simulink model "mDriverSimpleTest"  (R2019b)
settings: Solver=ode4  StartTime=0  StopTime=2474  FixedStep=0.01  MaxStep=.01  RelTol=1e-3
libraries: VsrLibDriver x1, VsrLibDriveCycleSrc x1, autolibshared x1
settings Model: DataDictionary=DdDriverLongTest.sldd  SimulationMode=accelerator  PauseTimes=70  Creator=9bt  LastModifiedBy=4qz

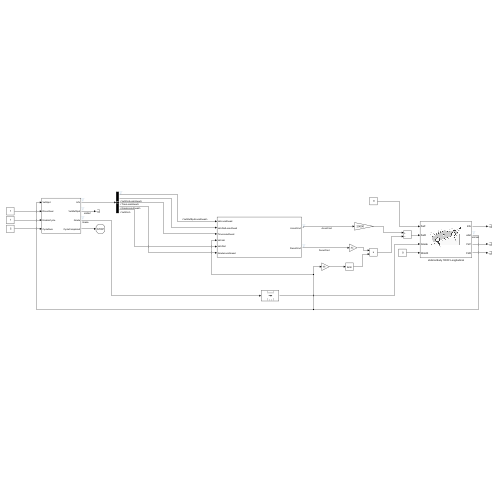
[thumbnail: Simulink's stored preview of the top-level diagram]
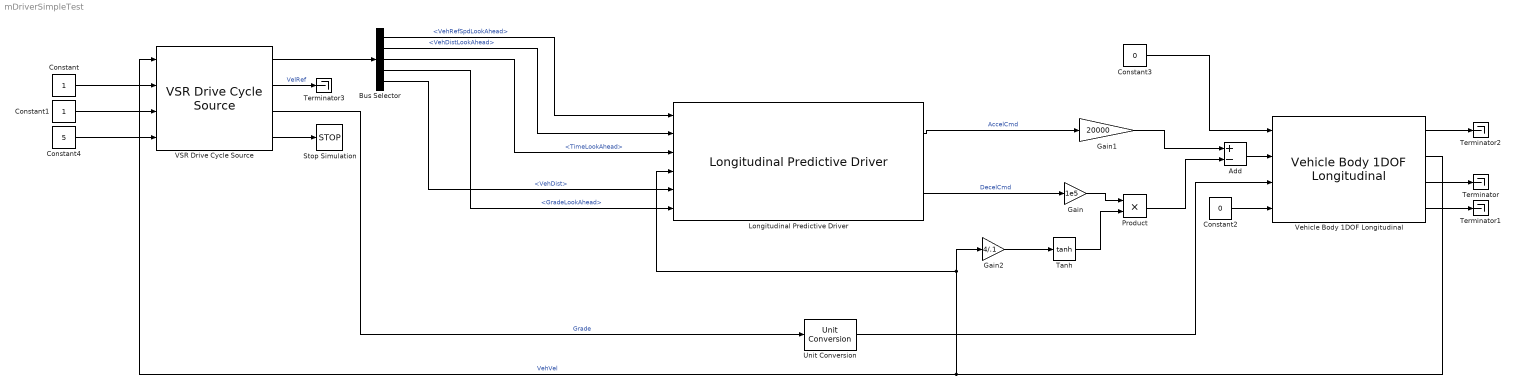
== system mDriverSimpleTest ==
  Add : Sum  Inputs=+-
  Bus Selector : BusSelector  OutputSignals=VehRefSpdLookAhead,VehDistLookAhead,TimeLookAhead,GradeLookAhead,VehDist
  Constant : Constant
  Constant1 : Constant
  Constant2 : Constant  Value=0
  Constant3 : Constant  Value=0
  Constant4 : Constant  Value=5
  Gain : Gain  Gain=1e5
  Gain1 : Gain  Gain=20000
  Gain2 : Gain  Gain=4/.1
  Longitudinal Predictive Driver : VsrLibDriver/Longitudinal Predictive Driver  VehMass=1500  aR=200  bR=2.5  cR=0.5  MaxAccelFrcSpdBpts=[ 10, 100 ]  MaxAccelFrcTbl=[ 10000, 10000 ]  AccelPdlBpts=[ 0, 1 ]  AccelPdlTbl=[ 0, 1 ]  BrakePdlBpts=[ 0, 1 ]  BrakeFrcTbl=[ 0, 1e5 ]  SmoothTimeAvg=.5  VelThresh=.1  PdlRateLimitWeight=.1  DistOptWeight=100  NumOptimIters=20  g=9.81
  Product : Product
  Stop Simulation : Stop
  Tanh : Trigonometry  Operator=tanh
  Terminator{,1..3} (4 alike) : Terminator
  Unit Conversion : UnitConversion
  VSR Drive Cycle Source : VsrLibDriveCycleSrc/VSR Drive Cycle Source  DistCompensationCheckbox=off  DriveCycleStructArray=VsrDriveCycleStructArray  TimeLookAhead=LookAheadTime
  Vehicle Body 1DOF Longitudinal : autolibshared/Vehicle Body 1DOF Longitudinal  VariantControl=SL  extFMode=off  extMMode=off  extTamb=off  wind3D=off  aMode=1  NF=2  NR=2  m=1500  a=1.4  b=1.8  h=.35  Cd=.3  Cl=0  Cpm=0  Af=4  x_o=0  xdot_o=0  Pabs=101325  T=273  g=9.81
  wires:
  Bus Selector/1 -> Longitudinal Predictive Driver/1  "<VehRefSpdLookAhead>"
  Constant2/1 -> Vehicle Body 1DOF Longitudinal/4
  Vehicle Body 1DOF Longitudinal/2 -> VSR Drive Cycle Source/1, Longitudinal Predictive Driver/4, Gain2/1  "VehVel"
  Vehicle Body 1DOF Longitudinal/3 -> Terminator/1
  Vehicle Body 1DOF Longitudinal/4 -> Terminator1/1
  Unit Conversion/1 -> Vehicle Body 1DOF Longitudinal/3
  VSR Drive Cycle Source/3 -> Unit Conversion/1  "Grade"
  Vehicle Body 1DOF Longitudinal/1 -> Terminator2/1
  Constant3/1 -> Vehicle Body 1DOF Longitudinal/1
  Add/1 -> Vehicle Body 1DOF Longitudinal/2
  Product/1 -> Add/2
  Gain1/1 -> Add/1
  Gain/1 -> Product/1
  Tanh/1 -> Product/2
  Gain2/1 -> Tanh/1
  Longitudinal Predictive Driver/1 -> Gain1/1  "AccelCmd"
  Longitudinal Predictive Driver/2 -> Gain/1  "DecelCmd"
  VSR Drive Cycle Source/2 -> Terminator3/1  "VelRef"
  VSR Drive Cycle Source/4 -> Stop Simulation/1
  VSR Drive Cycle Source/1 -> Bus Selector/1
  Constant1/1 -> VSR Drive Cycle Source/3
  Constant/1 -> VSR Drive Cycle Source/2
  Constant4/1 -> VSR Drive Cycle Source/4
  Bus Selector/2 -> Longitudinal Predictive Driver/2  "<VehDistLookAhead>"
  Bus Selector/3 -> Longitudinal Predictive Driver/3  "<TimeLookAhead>"
  Bus Selector/4 -> Longitudinal Predictive Driver/6  "<GradeLookAhead>"
  Bus Selector/5 -> Longitudinal Predictive Driver/5  "<VehDist>"
